simulink model "sf_framesync"  (R2015b)
settings: Solver=FixedStepDiscrete  SolverMode=SingleTasking  StartTime=0.0  StopTime=10000  RelTol=1e-3
PreLoadFcn:
  | frame_sync_param
values from neighbouring files (symbols this model uses):
  FrameSize = 32    [frame_sync_param.m]
  SyncCode = hex2dec('47')    [frame_sync_param.m]
  SyncSig = str2num(dec2bin(SyncCode,SyncCodeSize)')    [frame_sync_param.m]
libraries: dspsrcs4 x2, commrandsrc2 x1, commchan3 x1
settings Model: DataTypeOverride=Off  Creator=amatsumo  LastModifiedBy=amatsumo
settings DataIOCC: SaveFormat=Array  SaveOutput=off  SignalLogging=off  SaveTime=off
settings OptimizationCC: BlockReduction=off  ConditionallyExecuteInputs=off  DefaultParameterBehavior=Inlined
settings DebuggingCC: AlgebraicLoopMsg=error  SolverPrmCheckMsg=warning  SingleTaskRateTransMsg=error
settings HardwareCC: ProdBitPerPointer=32  ProdLargestAtomicFloat=None  ProdIntDivRoundTo=Undefined  ProdEndianess=Unspecified  ProdWordSize=32  ProdHWDeviceType=ASIC/FPGA->ASIC/FPGA  ProdEqTarget=off
settings GRTTargetCC: GeneratePreprocessorConditionals=Disable all
settings ConfigComp: CovModelRefEnable=Off  CovSFcnEnable=off

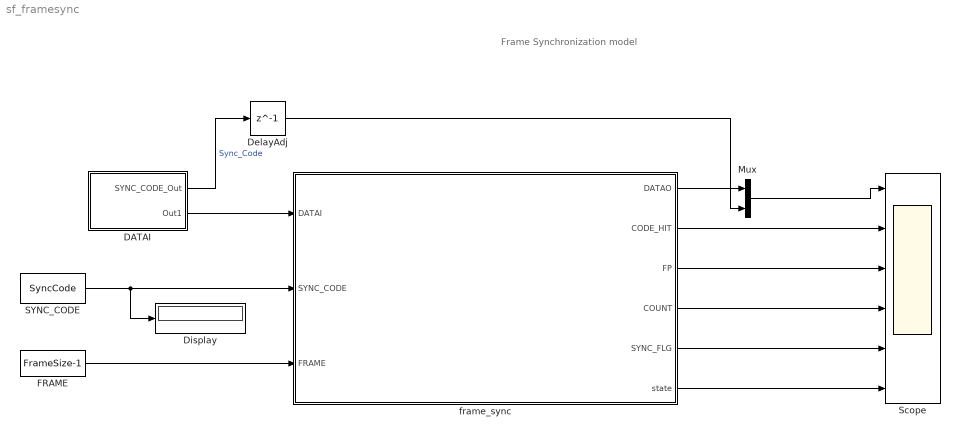
== system sf_framesync ==
  note: Frame Synchronization model
  DATAI : Subsystem
  DelayAdj : Delay  DelayLength=1
  Display : Display
      settings: Format=binary (Stored Integer)
  FRAME : Constant  Value=FrameSize-1  OutDataTypeStr=fixdt(0,8,0)  SampleTime=-1
  Mux : Mux  Inputs=2
  SYNC_CODE : Constant  Value=SyncCode  OutDataTypeStr=fixdt(0,8,0)  SampleTime=-1
  Scope : Scope  NumInputPorts=6
  frame_sync : Subsystem
  wires:
  SYNC_CODE/1 -> Display/1, frame_sync/2(SYNC_CODE)
  FRAME/1 -> frame_sync/3(FRAME)
  DATAI/2(Out1) -> frame_sync/1(DATAI)
  DATAI/1(SYNC_CODE_Out) -> DelayAdj/1  "Sync_Code"
  frame_sync/1(DATAO) -> Mux/1
  Mux/1 -> Scope/1
  frame_sync/2(CODE_HIT) -> Scope/2
  frame_sync/3(FP) -> Scope/3
  frame_sync/4(COUNT) -> Scope/4
  frame_sync/5(SYNC_FLG) -> Scope/5
  frame_sync/6(state) -> Scope/6
  DelayAdj/1 -> Mux/2

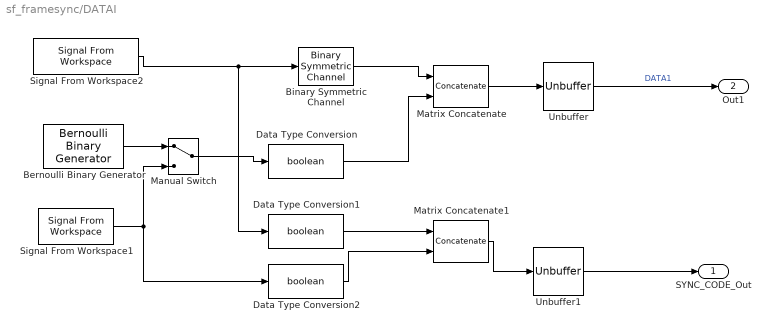
== system sf_framesync/DATAI ==
  Bernoulli Binary Generator : commrandsrc2/Bernoulli Binary Generator  P=0.5  seed=61  Ts=160/24  frameBased=on  sampPerFrame=24  orient=off  outDataType=double
  Binary Symmetric Channel : commchan3/Binary Symmetric Channel  P=0.04  s=366  E=off  outDtype=boolean
  Data Type Conversion : DataTypeConversion  OutDataTypeStr=boolean
  Data Type Conversion1 : DataTypeConversion  OutDataTypeStr=boolean
  Data Type Conversion2 : DataTypeConversion  OutDataTypeStr=boolean
  Manual Switch : ManualSwitch
  Matrix Concatenate : Concatenate  Mode=Multidimensional array
  Matrix Concatenate1 : Concatenate  Mode=Multidimensional array
  Signal From Workspace1 : dspsrcs4/Signal From Workspace  X=zeros(24,1)  Ts=160/24  nsamps=24  OutputAfterFinalValue=Cyclic repetition  ignoreOrWarnInputAndFrameLengths=off  OutputFrames=on
  Signal From Workspace2 : dspsrcs4/Signal From Workspace  X=SyncSig  Ts=160/(length(SyncSig))  nsamps=length(SyncSig)  OutputAfterFinalValue=Cyclic repetition  ignoreOrWarnInputAndFrameLengths=off  OutputFrames=on
  Unbuffer : Unbuffer  SampleBasedProcessing=Same as frame based
  Unbuffer1 : Unbuffer  SampleBasedProcessing=Same as frame based
  SYNC_CODE_Out : Outport
  Out1 : Outport  Port=2
  wires:
  Binary Symmetric Channel/1 -> Matrix Concatenate/1
  Data Type Conversion2/1 -> Matrix Concatenate1/2
  Manual Switch/1 -> Data Type Conversion/1
  Signal From Workspace1/1 -> Data Type Conversion2/1, Manual Switch/2
  Bernoulli Binary Generator/1 -> Manual Switch/1
  Data Type Conversion1/1 -> Matrix Concatenate1/1
  Unbuffer1/1 -> SYNC_CODE_Out/1
  Matrix Concatenate1/1 -> Unbuffer1/1
  Signal From Workspace2/1 -> Binary Symmetric Channel/1, Data Type Conversion1/1
  Data Type Conversion/1 -> Matrix Concatenate/2
  Matrix Concatenate/1 -> Unbuffer/1
  Unbuffer/1 -> Out1/1  "DATA1"

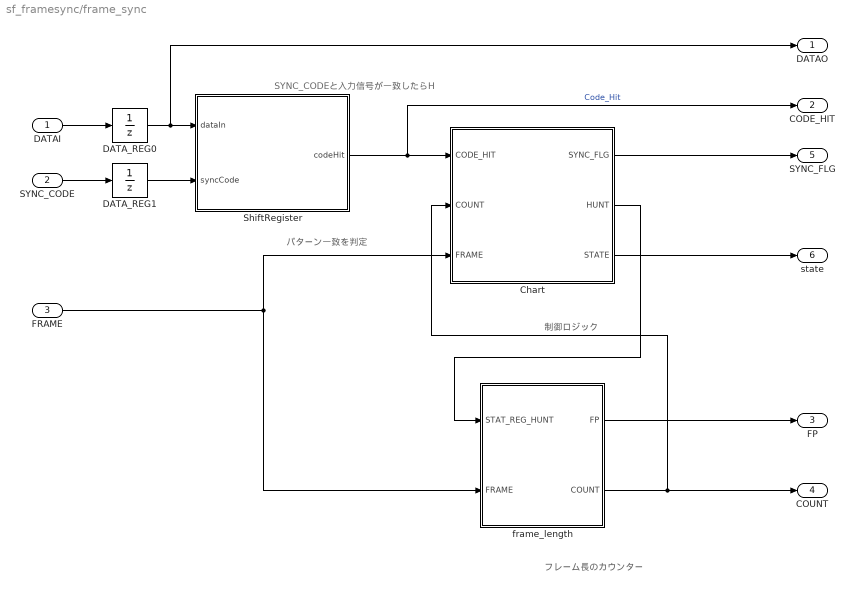
== system sf_framesync/frame_sync ==
  note: SYNC_CODEと入力信号が一致したらH
  note: フレーム長のカウンター
  note: 制御ロジック
  note: パターン一致を判定
  DATAI : Inport
  SYNC_CODE : Inport  Port=2
  FRAME : Inport  Port=3
  Chart : Stateflow chart  TreatAsAtomicUnit=on
  DATA_REG0 : UnitDelay  SampleTime=-1
  DATA_REG1 : UnitDelay  SampleTime=-1
  ShiftRegister : MATLAB Function  TreatAsAtomicUnit=on
  frame_length : Subsystem
      settings: MinAlgLoopOccurrences=on
  DATAO : Outport
  CODE_HIT : Outport  Port=2
  FP : Outport  Port=3
  COUNT : Outport  Port=4
  SYNC_FLG : Outport  Port=5
  state : Outport  Port=6
  wires:
  DATAI/1 -> DATA_REG0/1
  SYNC_CODE/1 -> DATA_REG1/1
  ShiftRegister/1(codeHit) -> Chart/1(CODE_HIT), CODE_HIT/1  "Code_Hit"
  DATA_REG1/1 -> ShiftRegister/2(syncCode)
  Chart/3(STATE) -> state/1
  frame_length/2(COUNT) -> Chart/2(COUNT), COUNT/1
  FRAME/1 -> frame_length/2(FRAME), Chart/3(FRAME)
  DATA_REG0/1 -> ShiftRegister/1(dataIn), DATAO/1
  frame_length/1(FP) -> FP/1
  Chart/2(HUNT) -> frame_length/1(STAT_REG_HUNT)
  Chart/1(SYNC_FLG) -> SYNC_FLG/1

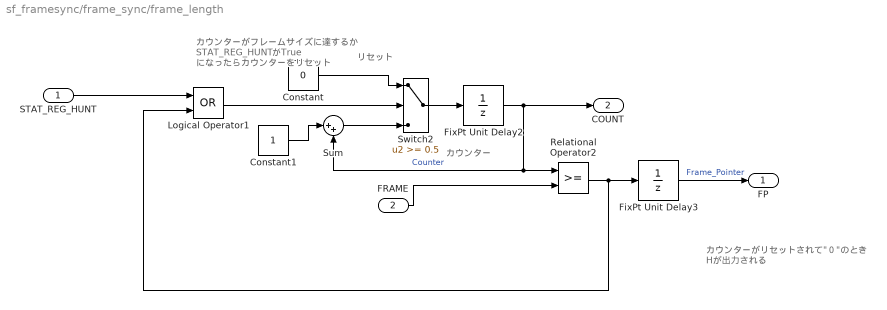
== system sf_framesync/frame_sync/frame_length ==
  note: カウンターがリセットされて"０"のとき
      | Hが出力される
  note: リセット
  note: カウンター
  note: カウンターがフレームサイズに達するか
      | STAT_REG_HUNTがTrue
      | になったらカウンターをリセット
  STAT_REG_HUNT : Inport
  FRAME : Inport  Port=2
  Constant : Constant  Value=0  OutDataTypeStr=uint8  SampleTime=-1
  Constant1 : Constant  OutDataTypeStr=fixdt(0,4,0)  SampleTime=-1
  FixPt Unit Delay2 : UnitDelay  SampleTime=-1
  FixPt Unit Delay3 : UnitDelay  SampleTime=-1
  Logical Operator1 : Logic  Operator=OR  AllPortsSameDT=off  OutDataTypeStr=boolean
  Relational Operator2 : RelationalOperator  OutDataTypeStr=boolean  ZeroCross=off
  Sum : Sum  Inputs=|++  OutDataTypeStr=fixdt(0,8,0)
  Switch2 : Switch  Threshold=0.5  ZeroCross=off
  FP : Outport
  COUNT : Outport  Port=2
  wires:
  Constant/1 -> Switch2/1
  Switch2/1 -> FixPt Unit Delay2/1
  Constant1/1 -> Sum/1
  Sum/1 -> Switch2/3
  FRAME/1 -> Relational Operator2/2
  Logical Operator1/1 -> Switch2/2
  FixPt Unit Delay2/1 -> COUNT/1, Relational Operator2/1, Sum/2  "Counter"
  Relational Operator2/1 -> FixPt Unit Delay3/1, Logical Operator1/2
  STAT_REG_HUNT/1 -> Logical Operator1/1
  FixPt Unit Delay3/1 -> FP/1  "Frame_Pointer"

== stateflow chart sf_framesync/frame_sync/Chart ==
  settings: stateMachineType=MOORE_MACHINE  initializeOutput=1
  state HUNT/
    SYNC_FLG = 0;
    HUNT = 1;
    STATE=1;
  note: 情報表示/Stateflowアニメーション/
      | で表示速度を調節可能
  state FOUND/
    SYNC_FLG = 0;
    HUNT = 0;
    STATE=2;
  state LOST/
    SYNC_FLG = 1;
    HUNT = 0;
    STATE=4;
  state SYNC/
    SYNC_FLG = 1;
    HUNT = 0;
    STATE=3;
  (default) -> HUNT
  HUNT -> FOUND : [CODE_HIT == 1]
  (junction 31) -> HUNT [order 2]
  (junction 27) -> HUNT [order 2]
  LOST -> (junction 31) : [COUNT == FRAME]
  FOUND -> (junction 27) : [COUNT == FRAME]
  (junction 31) -> SYNC [order 1] : [CODE_HIT == 1]
  (junction 27) -> SYNC [order 1] : [CODE_HIT == 1]
  SYNC -> LOST : [COUNT == FRAME &&...
      |  CODE_HIT == 0]
  data: CODE_HIT input; COUNT input; SYNC_FLG output boolean; HUNT output boolean; FRAME input; STATE output uint8

== matlab function sf_framesync/frame_sync/ShiftRegister ==
  settings: fimath=|
      | fimath(...
      | 'RoundMode', 'floor',...
      | 'OverflowMode', 'wrap',...
      | 'ProductMode', 'FullPrecision', 'ProductWordLength', 32,...
      | 'SumMode', 'FullPrecision', 'SumWordLength', 32,...
      | 'CastBeforeSum', true)
  data: dataIn input boolean; codeHit output fixdt(0,1,0); syncCode input
function codeHit = fcn(dataIn, syncCode)

persistent u_d;
if isempty(u_d)
    u_d = fi(zeros(1,8), 0,8,0);
end

d1 = uint8(dataIn);
d2 = uint8(bitshift(u_d(1),1));
d3 = uint8(bitshift(u_d(2),2));
d4 = uint8(bitshift(u_d(3),3));
d5 = uint8(bitshift(u_d(4),4));
d6 = uint8(bitshift(u_d(5),5));
d7 = uint8(bitshift(u_d(6),6));
d8 = uint8(bitshift(u_d(7),7));

u_d = [dataIn, u_d(1), u_d(2), u_d(3), u_d(4), u_d(5), u_d(6), u_d(7)];

tmp = bitxor(d1, d2);
tmp = bitxor(tmp, d3);
tmp = bitxor(tmp, d4);
tmp = bitxor(tmp, d5);
tmp = bitxor(tmp, d6);
tmp = bitxor(tmp, d7);
tmp = bitxor(tmp, d8);

codeHit = fi((syncCode == tmp), 0,1, 0);
